simulink model "surge_tank_level_sim"  (R2021b)
settings: Solver=VariableStepAuto  StartTime=0.0  StopTime=5000  MaxStep=0.1  RelTol=1e-3  EnableMultiTasking=on
InitFcn:
  | load("mpcobj.mat")
StopFcn:
  | addpath("~/ml-plot-utils")
  | 
  | figure(1); clf
  | u_labels = ["$u(k)$" "$p(k)$"];
  | make_iorplot(y, t, [u p], r, u_labels)
  | sp1 = subplot(2,1,1);
  | ylim(sp1,axes_limits_with_margin(y, 0.1, [0 100]))
  | 
  | figure(2); clf
  | u_labels = ["$u(k)$" "$p(k)$"];
  | make_iorplot(y1, t, [u1 p], r, u_labels)
  | sp1 = subplot(2,1,1);
  | ylim(sp1,axes_limits_with_margin(y, 0.1, [0 100]))
  | 
  | figure(3); clf
  | u_labels = ["$u(k)$" "$p(k)$"];
  | make_iorplot(y2, t, [u2 p], r, u_labels)
  | sp1 = subplot(2,1,1);
  | ylim(sp1,axes_limits_with_margin(y, 0.1, [0 100]))
  | 
  | figure(4); clf
  | u_labels = ["$u(k)$" "$p(k)$"];
  | make_iorplot(y3, t, [u3 p], r, u_labels)
  | sp1 = subplot(2,1,1);
  | ylim(sp1,[0 100])
  | yline(15, '--', 'Parent', sp1)
  | yline(85, '--', 'Parent', sp1)
  | labels = sp1.Legend.String;
  | labels(3:4) = {'$y_{min}$', '$y_{max}$'};
  | set(sp1.Legend, 'String', labels)
  | 
  | figure(5); clf
  | u_labels = ["$u(k)$" "$p(k)$"];
  | make_iorplot(y4, t, [u4 p], r, u_labels)
  | sp1 = subplot(2,1,1);
  | ylim(sp1,[0 100])
  | yline(15, '--', 'Parent', sp1)
  | yline(85, '--', 'Parent', sp1)
  | labels = sp1.Legend.String;
  | labels(3:4) = {'$y_{min}$', '$y_{max}$'};
  | set(sp1.Legend, 'String', labels)
  | 
  | figure(6); clf
  | u_labels = ["$u(k)$" "$p(k)$"];
  | make_iorplot(y5, t, [u5 p], r, u_labels)
  | sp1 = subplot(2,1,1);
  | ylim(sp1,[0 100])
  | yline(15, '--', 'Parent', sp1)
  | yline(85, '--', 'Parent', sp1)
  | labels = sp1.Legend.String;
  | labels(3:4) = {'$y_{min}$', '$y_{max}$'};
  | set(sp1.Legend, 'String', labels)
  | 
  | figure(7); clf
  | u_labels = ["$u(k)$" "$p(k)$"];
  | make_iorplot(y6, t, [u6 p], r, u_labels)
  | sp1 = subplot(2,1,1);
  | ylim(sp1,[0 100])
  | yline(15,'--', 'Parent', sp1)
  | yline(85, '--', 'Parent', sp1)
  | labels = sp1.Legend.String;
  | labels(3:4) = {'$y_{min}$', '$y_{max}$'};
  | set(sp1.Legend, 'String', labels)
  | 
  | figure(7); clf
  | u_labels = ["$u(k)$" "$p(k)$"];
  | make_iorplot(y6, t, [u6 p], r, u_labels)
  | sp1 = subplot(2,1,1);
  | ylim(sp1,[0 100])
  | yline(15,'--', 'Parent', sp1)
  | yline(85, '--', 'Parent', sp1)
  | labels = sp1.Legend.String;
  | labels(3:4) = {'$y_{min}$', '$y_{max}$'};
  | set(sp1.Legend, 'String', labels)
  | 
  | figure(8); clf
  | u_labels = ["$u(k)$" "$p(k)$"];
  | make_iorplot(y7, t, [u7 p], r, u_labels)
  | sp1 = subplot(2,1,1);
  | ylim(sp1,[0 100])
  | yline(15,'--', 'Parent', sp1)
  | yline(85, '--', 'Parent', sp1)
  | labels = sp1.Legend.String;
  | labels(3:4) = {'$y_{min}$', '$y_{max}$'};
  | set(sp1.Legend, 'String', labels)
  | 
  | figure(9); clf
  | u_labels = ["$u(k)$" "$p(k)$"];
  | make_iorplot(y8, t, [u8 p], r, u_labels)
  | sp1 = subplot(2,1,1);
  | ylim(sp1,[0 100])
  | yline(15,'--', 'Parent', sp1)
  | yline(85, '--', 'Parent', sp1)
  | labels = sp1.Legend.String;
  | labels(3:4) = {'$y_{min}$', '$y_{max}$'};
  | set(sp1.Legend, 'String', labels)
undefined symbols (not defined in the file or in its folder): DiscIntNeverNeededParam
libraries: simulink x10, dspstat3 x3, mpclib x1
settings Model: PacingRate=10  Creator=Eric  LastModifiedBy=billtubbs
settings SolverCC: ZeroCrossAlgorithm=Adaptive  AlgebraicLoopSolver=TrustRegion
settings DataIOCC: LimitDataPoints=on  SaveFormat=StructureWithTime  SignalLoggingSaveFormat=ModelDataLogs  SaveTime=off  ReturnWorkspaceOutputs=off
settings OptimizationCC: ExpressionDepthLimit=2147483647  LifeSpan=inf
settings DebuggingCC: AlgebraicLoopMsg=none  UnderspecifiedInitializationDetection=Classic  MergeDetectMultiDrivingBlocksExec=none  IgnoredZcDiagnostic=none  FcnCallInpInsideContextMsg=warning  UnconnectedInputMsg=none  UnconnectedOutputMsg=none  UnconnectedLineMsg=none  StateNameClashWarn=warning  SFUnexpectedBacktrackingDiag=warning  SFNoUnconditionalDefaultTransitionDiag=warning  SFExecutionAtInitializationDiag=none  SFMachineParentedDataDiag=warning  ArithmeticOperatorsInVariantConditions=warning
settings HardwareCC: ProdBitPerPointer=32  ProdBitPerSizeT=32  ProdBitPerPtrDiffT=32  ProdLargestAtomicFloat=None  ProdIntDivRoundTo=Undefined  ProdEndianess=Unspecified  ProdWordSize=32  ProdHWDeviceType=32-bit Generic
settings ModelReferenceCC: PropagateSignalLabelsOutOfModel=off
settings SFSimCC: SimUseLocalCustomCode=off  CustomCodeUndefinedFunction=UseInterfaceOnly
settings RTWCC: RTWUseLocalCustomCode=off
settings CodeAppCC: StateflowObjectComments=on
settings GRTTargetCC: TargetLangStandard=C89/C90 (ANSI)  CombineOutputUpdateFcns=off  GRTInterface=on
settings ConfigComp: CovMetricSettings=dw  CovSaveCumulativeToWorkspaceVar=on  CovSaveSingleToWorkspaceVar=on  CovExternalEMLEnable=off  CovSFcnEnable=off

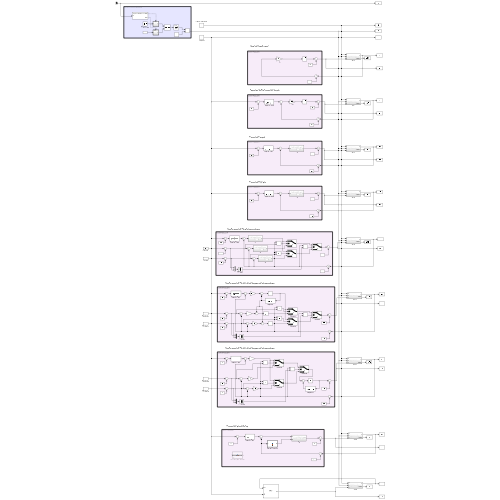
[thumbnail: Simulink's stored preview of the top-level diagram]
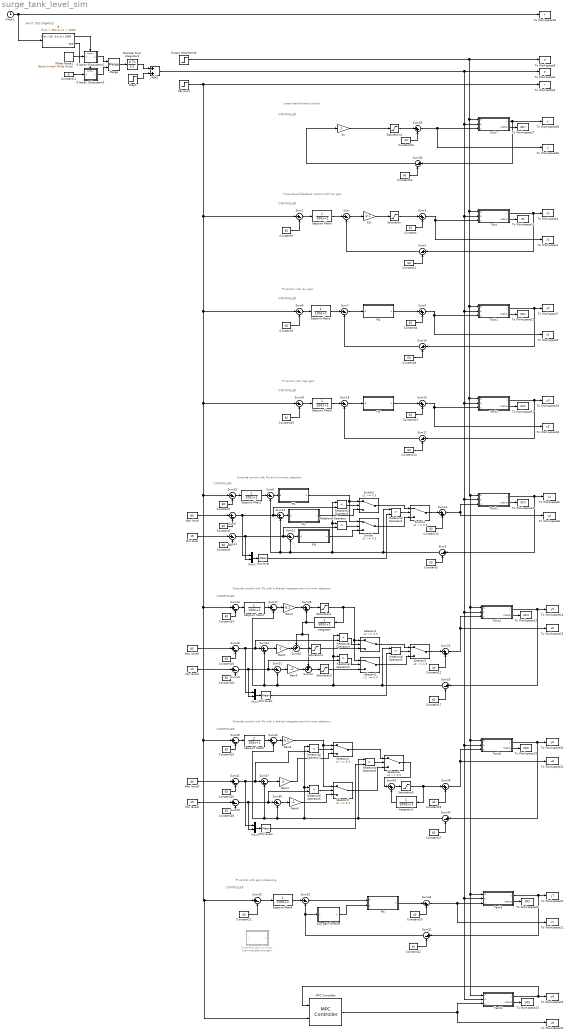
== system surge_tank_level_sim ==
  note: Proportional feedback control with low gain
  note: Override control with PIs and min-max selectors
  note: CONTROLLER
  note: CONTROLLER
  note: INPUT DISTURBANCE
  note: PI control with low gain
  note: CONTROLLER
  note: CONTROLLER
  note: PI control with high gain
  note: CONTROLLER
  note: Override control with PIs with a shared integrator and min-max selectors
  note: PI control with gain scheduling
  note: CONTROLLER
  note: CONTROLLER
  note: Linear feed-forward control
  note: CONTROLLER
  note: Override control with PIs with a shared integrator and min-max selectors
  Add1 : Sum
  Clock1 : Clock
  Constant{,4,10,12..13,20,23,25} (8 alike) : Constant  Value=40
  Constant{1..3,5..9,14..19,21..22,24,26..29} (21 alike) : Constant  Value=60
  Constant11 : Constant  Value=0
  Discrete-Time Integrator1 : DiscreteIntegrator  gainval=1  SampleTime=-1  ICPrevOutput=DiscIntNeverNeededParam  ICPrevScaledInput=DiscIntNeverNeededParam
  Exp gain function : MATLAB Function  TreatAsAtomicUnit=on
  Gain{1,3..4,6} (4 alike) : Gain  Gain=-2
  Gain2 : Gain  Gain=-0.1
  Gain5 : Gain  Gain=-0.1
  If : If  IfExpression=u1 > 500 & u1 < 1000
  If Action Subsystem2 : Subsystem  TreatAsAtomicUnit=on
  If Action Subsystem3 : Subsystem  TreatAsAtomicUnit=on
  Integrator : TransferFcn  Numerator=1  Denominator=[500 1]
  Integrator1 : TransferFcn  Numerator=1  Denominator=[1000 1]
  Kc : Gain
  Kc1 : Gain  Gain=-0.1
  MPC Controller : mpclib/MPC Controller  mpcobj=mpcobj  x0=[]  is_multiple=0  enable_value=0  return_u0=off  updateMPCinCallerWorkspace=on  md_inport=off  mv_inport=off  uref_inport=off  return_cost=off  return_mvseq=off  return_qpstatus=off  return_xseq=off  return_state=off  return_ovseq=off  state_inport=off  umin_inport=off  umax_inport=off  ymin_inport=off  ymax_inport=off  cc_inport=off  ywt_inport=off  uwt_inport=off  duwt_inport=off  rhoeps_inport=off  pm_inport=off  MaximumP=10  HorizonChoice=FixedHorizon  n_ts=5  n_p=200  n_mv=1  n_md=0  n_ud=1  n_mo=1  n_uo=0  BlockDataType=double  SampleTimeInherited=off  switch_inport=off
  Max level : Constant  Value=85
  Max level1 : Constant  Value=85
  Max level2 : Constant  Value=85
  Merge : Merge
  Mid level : dspstat3/Mean  run=off  InputProcessing=Columns as channels (frame based)  reset_popup=None  directionMode=Entire input  dimension=1  roiEnable=off  roiType=Rectangles  roiPortion=Entire ROI  roiOutput=Individual statistics for each ROI  roiFlag=off  roundingMode=Floor  overflowMode=off  outputDataTypeStr=Inherit: Same as accumulator  outputMin=[]  outputMax=[]  outputLastDataTypeStr=Inherit: Same as accumulator
  Mid level1 : dspstat3/Mean  run=off  InputProcessing=Columns as channels (frame based)  reset_popup=None  directionMode=Entire input  dimension=1  roiEnable=off  roiType=Rectangles  roiPortion=Entire ROI  roiOutput=Individual statistics for each ROI  roiFlag=off  roundingMode=Floor  overflowMode=off  outputDataTypeStr=Inherit: Same as accumulator  outputMin=[]  outputMax=[]  outputLastDataTypeStr=Inherit: Same as accumulator
  Mid level2 : dspstat3/Mean  run=off  InputProcessing=Columns as channels (frame based)  reset_popup=None  directionMode=Entire input  dimension=1  roiEnable=off  roiType=Rectangles  roiPortion=Entire ROI  roiOutput=Individual statistics for each ROI  roiFlag=off  roundingMode=Floor  overflowMode=off  outputDataTypeStr=Inherit: Same as accumulator  outputMin=[]  outputMax=[]  outputLastDataTypeStr=Inherit: Same as accumulator
  Min level : Constant  Value=15
  Min level1 : Constant  Value=15
  Min level2 : Constant  Value=15
  Mux1 : Mux  Inputs=2
  Mux2 : Mux  Inputs=2
  Mux3 : Mux  Inputs=2
  Output disturbance : Step  After=0  SampleTime=0
  PI1 : Subsystem
  PI2 : Subsystem
  PI3 : Subsystem
  PI4 : Subsystem
  PI5 : Subsystem
  PI6 : Subsystem
  Quadratic gain function : MATLAB Function  Commented=through  TreatAsAtomicUnit=on
  Relational Operator{,2..3,5..6,8} (6 alike) : RelationalOperator  Operator=>  OutDataTypeStr=boolean  RndMeth=Nearest
  Relational Operator1 : RelationalOperator  Operator=<  OutDataTypeStr=boolean  RndMeth=Nearest
  Relational Operator4 : RelationalOperator  Operator=<  OutDataTypeStr=boolean  RndMeth=Nearest
  Relational Operator7 : RelationalOperator  Operator=<  OutDataTypeStr=boolean  RndMeth=Nearest
  Saturation{,1..5} (6 alike) : Saturate  UpperLimit=60  LowerLimit=-40
  Selector{1..6} (6 alike) : Switch  Threshold=0.5
  Set point : Step  Time=100  Before=60  After=50  SampleTime=0
  Setpoint filter{0..6} (7 alike) : TransferFcn  Denominator=[100 1]
  Step1 : Step  Time=900  After=10  SampleTime=0
  Sum{,1..2,4..8,10..13,15..19,21..22,24..27,29..33,36..37,39..42} (34 alike) : Sum  Inputs=|+-
  Sum{3,9,14,20,23,28,34..35,38,43} (10 alike) : Sum  Inputs=|++
  Sum44 : Sum  Inputs=++|
  Sum45 : Sum  Inputs=++|
  Switch : Switch  Threshold=0.5
  Switch1 : Switch  Threshold=0.5
  Switch2 : Switch  Threshold=0.5
  Tank : Subsystem
  Tank1 : Subsystem
  Tank2 : Subsystem
  Tank3 : Subsystem
  Tank4 : Subsystem
  Tank5 : Subsystem
  Tank6 : Subsystem
  Tank7 : Subsystem
  Tank8 : Subsystem
  To Workspace1 : ToWorkspace  VariableName=u1  SampleTime=1
  To Workspace10 : ToWorkspace  VariableName=OF  SaveFormat=Timeseries  SampleTime=-1
  To Workspace11 : ToWorkspace  VariableName=OF1  SaveFormat=Timeseries  SampleTime=-1
  To Workspace12 : ToWorkspace  VariableName=OF3  SaveFormat=Timeseries  SampleTime=-1
  To Workspace13 : ToWorkspace  VariableName=OF4  SaveFormat=Timeseries  SampleTime=-1
  To Workspace14 : ToWorkspace  VariableName=y5  SampleTime=1
  To Workspace15 : ToWorkspace  VariableName=u5  SampleTime=1
  To Workspace16 : ToWorkspace  VariableName=t  SampleTime=1
  To Workspace17 : ToWorkspace  VariableName=OF2  SaveFormat=Timeseries  SampleTime=-1
  To Workspace18 : ToWorkspace  VariableName=u3  SampleTime=1
  To Workspace19 : ToWorkspace  VariableName=y3  SampleTime=1
  To Workspace2 : ToWorkspace  VariableName=y1  SampleTime=1
  To Workspace20 : ToWorkspace  VariableName=OF5  SaveFormat=Timeseries  SampleTime=-1
  To Workspace21 : ToWorkspace  VariableName=u7  SampleTime=1
  To Workspace22 : ToWorkspace  VariableName=y7  SampleTime=1
  To Workspace23 : ToWorkspace  VariableName=OF6  SaveFormat=Timeseries  SampleTime=-1
  To Workspace24 : ToWorkspace  VariableName=u8  SampleTime=1
  To Workspace25 : ToWorkspace  VariableName=y8  SampleTime=1
  To Workspace26 : ToWorkspace  VariableName=u  SampleTime=1
  To Workspace27 : ToWorkspace  VariableName=OF7  SaveFormat=Timeseries  SampleTime=-1
  To Workspace28 : ToWorkspace  VariableName=y  SampleTime=1
  To Workspace29 : ToWorkspace  VariableName=OF8  SaveFormat=Timeseries  SampleTime=-1
  To Workspace3 : ToWorkspace  VariableName=r  SampleTime=1
  To Workspace30 : ToWorkspace  VariableName=y6  SampleTime=1
  To Workspace31 : ToWorkspace  VariableName=u6  SampleTime=1
  To Workspace4 : ToWorkspace  VariableName=p  SampleTime=1
  To Workspace5 : ToWorkspace  VariableName=u2  SampleTime=1
  To Workspace6 : ToWorkspace  VariableName=y4  SampleTime=1
  To Workspace7 : ToWorkspace  VariableName=y2  SampleTime=1
  To Workspace8 : ToWorkspace  VariableName=u4  SampleTime=1
  To Workspace9 : ToWorkspace  VariableName=d  SampleTime=1
  White Noise1 : simulink/Sources/Band-Limited White Noise  Cov=0.1  Ts=1  seed=[10000]
  wires:
  Setpoint filter2/1 -> Sum6/1
  Sum2/1 -> Relational Operator1/1, Relational Operator/1, Sum12/2, Sum13/2, Sum6/2, Relational Operator2/1
  Sum6/1 -> PI1/1(e)
  PI1/1(u) -> Switch/1, Switch1/1
  Sum5/1 -> Relational Operator1/2, Sum13/1, Mux1/1
  Relational Operator1/1 -> Switch1/2
  Sum13/1 -> PI2/1(e)
  Sum12/1 -> PI3/1(e)
  Sum11/1 -> Relational Operator/2, Sum12/1, Mux1/2
  Relational Operator/1 -> Switch/2
  PI2/1(u) -> Switch1/3
  PI3/1(u) -> Switch/3
  Switch1/1 -> Switch2/1
  Switch/1 -> Switch2/3
  Relational Operator2/1 -> Switch2/2
  Mid level/1 -> Relational Operator2/2
  Constant2/1 -> Sum5/2
  Max level/1 -> Sum5/1
  Constant5/1 -> Sum11/2
  Min level/1 -> Sum11/1
  Sum15/1 -> Setpoint filter2/1
  Constant7/1 -> Sum15/2
  Mux1/1 -> Mid level/1
  Sum4/1 -> Sum/2
  Constant6/1 -> Sum1/2
  Sum3/1 -> To Workspace1/1, Tank/3(u)
  Tank/1(y) -> Sum4/1, To Workspace2/1
  Tank/2(status) -> To Workspace10/1
  Constant1/1 -> Sum4/2
  Constant/1 -> Sum3/2
  Sum/1 -> Kc1/1
  Saturation/1 -> Sum3/1
  Constant3/1 -> Sum2/2
  Sum14/1 -> Tank2/3(u), To Workspace8/1
  Tank2/2(status) -> To Workspace12/1
  Tank2/1(y) -> Sum2/1, To Workspace6/1
  Kc1/1 -> Saturation/1
  Sum8/1 -> Setpoint filter1/1
  Tank1/1(y) -> Sum10/1, To Workspace7/1
  Sum7/1 -> PI4/1(e)
  PI4/1(u) -> Sum9/1
  Constant8/1 -> Sum10/2
  Setpoint filter1/1 -> Sum7/1
  Tank1/2(status) -> To Workspace11/1
  Sum9/1 -> Tank1/3(u), To Workspace5/1
  Constant4/1 -> Sum9/2
  Constant9/1 -> Sum8/2
  If/1 -> If Action Subsystem2/Action
  If/2 -> If Action Subsystem3/Action
  Clock1/1 -> If/1, To Workspace16/1
  If Action Subsystem2/1(Out1) -> Merge/1
  If Action Subsystem3/1(Out1) -> Merge/2
  White Noise1/1 -> If Action Subsystem2/1(In1)
  Constant11/1 -> If Action Subsystem3/1(In1)
  Discrete-Time Integrator1/1 -> Add1/1
  Step1/1 -> Add1/2
  Merge/1 -> Discrete-Time Integrator1/1
  Constant10/1 -> Sum14/2
  Switch2/1 -> Sum14/1
  Sum1/1 -> Setpoint filter0/1
  Setpoint filter0/1 -> Sum/1
  Sum10/1 -> Sum7/2
  Tank3/1(y) -> Sum17/1, To Workspace19/1
  Add1/1 -> Tank3/2(p), Tank4/2(p), Tank8/2(p), Tank5/2(p), Tank6/2(p), Tank2/2(p), Tank1/2(p), Tank/2(p), Tank7/2(p), To Workspace4/1
  PI5/1(u) -> Sum20/1
  Constant14/1 -> Sum17/2
  Constant15/1 -> Sum19/2
  Sum18/1 -> PI5/1(e)
  Sum20/1 -> Tank3/3(u), To Workspace18/1
  Constant13/1 -> Sum20/2
  Output disturbance/1 -> Tank/1(d), Tank3/1(d), Tank4/1(d), Tank8/1(d), Tank5/1(d), Tank6/1(d), Tank2/1(d), Tank1/1(d), Tank7/1(d), To Workspace9/1
  Sum17/1 -> Sum18/2
  Tank3/2(status) -> To Workspace17/1
  Sum19/1 -> Setpoint filter5/1
  Sum23/1 -> To Workspace15/1, Tank4/3(u)
  Mux2/1 -> Mid level1/1
  Constant16/1 -> Sum26/2
  Tank4/2(status) -> To Workspace13/1
  Selector1/1 -> Selector3/1
  Selector2/1 -> Selector3/3
  Saturation2/1 -> Selector1/3
  Sum26/1 -> Relational Operator4/2, Sum22/1, Mux2/1
  Constant18/1 -> Sum16/2
  Saturation3/1 -> Selector2/3
  Constant12/1 -> Sum23/2
  Constant17/1 -> Sum25/2
  Sum25/1 -> Sum27/2, Sum22/2, Sum21/2, Relational Operator3/1, Relational Operator4/1, Relational Operator5/1
  Relational Operator3/1 -> Selector2/2
  Setpoint filter3/1 -> Sum27/1
  Max level1/1 -> Sum26/1
  Constant19/1 -> Sum24/2
  Min level1/1 -> Sum16/1
  Mid level1/1 -> Relational Operator5/2
  Relational Operator5/1 -> Selector3/2
  Gain2/1 -> Sum28/1
  Tank4/1(y) -> Sum25/1, To Workspace14/1
  Sum24/1 -> Setpoint filter3/1
  Relational Operator4/1 -> Selector1/2
  Sum16/1 -> Sum21/1, Relational Operator3/2, Mux2/2
  Sum27/1 -> Gain2/1
  Gain1/1 -> Sum45/2
  Gain3/1 -> Sum44/2
  Sum22/1 -> Gain1/1
  Constant20/1 -> Sum34/2
  PI6/1(u) -> Sum34/1
  Tank5/2(status) -> To Workspace20/1
  Tank5/1(y) -> Sum31/1, To Workspace22/1
  Sum34/1 -> To Workspace21/1, Tank5/3(u)
  Sum33/1 -> Setpoint filter4/1
  Sum31/1 -> Sum32/2, Exp gain function/1(y)
  Constant21/1 -> Sum33/2
  Constant22/1 -> Sum31/2
  Sum32/1 -> PI6/1(e)
  Setpoint filter4/1 -> Sum32/1
  Exp gain function/1(K) -> PI6/2(K)
  Tank6/2(status) -> To Workspace23/1
  Tank6/1(y) -> MPC Controller/1, To Workspace25/1
  MPC Controller/1 -> To Workspace24/1, Tank6/3(u)
  Tank7/2(status) -> To Workspace27/1
  Kc/1 -> Saturation4/1
  Sum35/1 -> To Workspace26/1, Tank7/3(u)
  Tank7/1(y) -> Sum36/1, To Workspace28/1
  Constant24/1 -> Sum36/2
  Constant23/1 -> Sum35/2
  Saturation4/1 -> Sum35/1
  Sum36/1 -> Kc/1
  Setpoint filter5/1 -> Sum18/1
  Sum28/1 -> Saturation1/1
  Saturation1/1 -> Integrator/1, Selector1/1, Selector2/1
  Integrator/1 -> Sum44/1, Sum45/1, Sum28/2
  Sum21/1 -> Gain3/1
  Tank8/2(status) -> To Workspace29/1
  Sum37/1 -> Gain4/1
  Set point/1 -> Sum1/1, Sum19/1, Sum15/1, Sum24/1, Sum39/1, MPC Controller/2, Sum33/1, Sum8/1, To Workspace3/1
  Sum40/1 -> Sum42/2, Sum37/2, Sum30/2, Relational Operator7/1, Relational Operator6/1, Relational Operator8/1
  Selector5/1 -> Selector6/3
  Sum41/1 -> Relational Operator7/2, Sum37/1, Mux3/1
  Relational Operator7/1 -> Selector4/2
  Gain4/1 -> Selector4/3
  Sum42/1 -> Gain5/1
  Gain6/1 -> Selector5/3
  Constant28/1 -> Sum29/2
  Constant27/1 -> Sum40/2
  Constant29/1 -> Sum39/2
  Mid level2/1 -> Relational Operator8/2
  Max level2/1 -> Sum41/1
  Gain5/1 -> Selector5/1, Selector4/1
  Constant25/1 -> Sum38/2
  Setpoint filter6/1 -> Sum42/1
  Sum29/1 -> Sum30/1, Relational Operator6/2, Mux3/2
  Min level2/1 -> Sum29/1
  Sum38/1 -> To Workspace31/1, Tank8/3(u)
  Tank8/1(y) -> Sum40/1, To Workspace30/1
  Mux3/1 -> Mid level2/1
  Sum39/1 -> Setpoint filter6/1
  Relational Operator6/1 -> Selector5/2
  Selector6/1 -> Sum43/1
  Selector4/1 -> Selector6/1
  Sum43/1 -> Saturation5/1
  Saturation5/1 -> Sum38/1, Integrator1/1
  Relational Operator8/1 -> Selector6/2
  Integrator1/1 -> Sum43/2
  Constant26/1 -> Sum41/2
  Sum30/1 -> Gain6/1
  Selector3/1 -> Sum23/1
  Sum45/1 -> Saturation2/1
  Sum44/1 -> Saturation3/1

== system surge_tank_level_sim/If Action Subsystem2 ==
  In1 : Inport
  Action Port : ActionPort  ActionPortLabel=if(u1 > 500 & u1 < 1000)
  Out1 : Outport
  wires:
  In1/1 -> Out1/1

== system surge_tank_level_sim/If Action Subsystem3 ==
  In1 : Inport
  Action Port : ActionPort  ActionPortLabel=else
  Out1 : Outport
  wires:
  In1/1 -> Out1/1

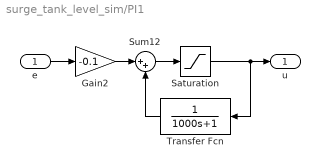
== system surge_tank_level_sim/PI1 ==
  e : Inport
  Gain2 : Gain  Gain=-0.1
  Saturation : Saturate  UpperLimit=60  LowerLimit=-40
  Sum12 : Sum  Inputs=|++
  Transfer Fcn : TransferFcn  Numerator=1  Denominator=[1000 1]
  u : Outport
  wires:
  e/1 -> Gain2/1
  Transfer Fcn/1 -> Sum12/2
  Gain2/1 -> Sum12/1
  Sum12/1 -> Saturation/1
  Saturation/1 -> Transfer Fcn/1, u/1

== system surge_tank_level_sim/PI2 ==
  e : Inport
  Gain2 : Gain  Gain=-2
  Saturation : Saturate  UpperLimit=60  LowerLimit=-40
  Sum12 : Sum  Inputs=|++
  Transfer Fcn : TransferFcn  Numerator=1  Denominator=[40 1]
  u : Outport
  wires:
  e/1 -> Gain2/1
  Transfer Fcn/1 -> Sum12/2
  Gain2/1 -> Sum12/1
  Sum12/1 -> Saturation/1
  Saturation/1 -> Transfer Fcn/1, u/1

== system surge_tank_level_sim/PI3 ==
  e : Inport
  Gain2 : Gain  Gain=-2
  Saturation : Saturate  UpperLimit=60  LowerLimit=-40
  Sum12 : Sum  Inputs=|++
  Transfer Fcn : TransferFcn  Numerator=1  Denominator=[40 1]
  u : Outport
  wires:
  e/1 -> Gain2/1
  Transfer Fcn/1 -> Sum12/2
  Gain2/1 -> Sum12/1
  Sum12/1 -> Saturation/1
  Saturation/1 -> Transfer Fcn/1, u/1

== system surge_tank_level_sim/PI4 ==
  e : Inport
  Gain2 : Gain  Gain=-0.1
  Saturation : Saturate  UpperLimit=60  LowerLimit=-40
  Sum12 : Sum  Inputs=|++
  Transfer Fcn : TransferFcn  Numerator=1  Denominator=[1000 1]
  u : Outport
  wires:
  e/1 -> Gain2/1
  Transfer Fcn/1 -> Sum12/2
  Gain2/1 -> Sum12/1
  Sum12/1 -> Saturation/1
  Saturation/1 -> Transfer Fcn/1, u/1

== system surge_tank_level_sim/PI5 ==
  e : Inport
  Gain2 : Gain  Gain=-2
  Saturation : Saturate  UpperLimit=60  LowerLimit=-40
  Sum12 : Sum  Inputs=|++
  Transfer Fcn : TransferFcn  Numerator=1  Denominator=[40 1]
  u : Outport
  wires:
  e/1 -> Gain2/1
  Transfer Fcn/1 -> Sum12/2
  Gain2/1 -> Sum12/1
  Sum12/1 -> Saturation/1
  Saturation/1 -> Transfer Fcn/1, u/1

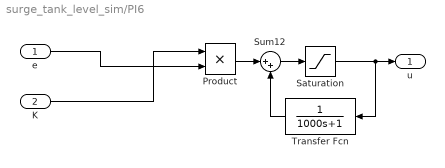
== system surge_tank_level_sim/PI6 ==
  e : Inport
  K : Inport  Port=2
  Product : Product
  Saturation : Saturate  UpperLimit=60  LowerLimit=-40
  Sum12 : Sum  Inputs=|++
  Transfer Fcn : TransferFcn  Numerator=1  Denominator=[1000 1]
  u : Outport
  wires:
  e/1 -> Product/2
  Transfer Fcn/1 -> Sum12/2
  Product/1 -> Sum12/1
  Sum12/1 -> Saturation/1
  Saturation/1 -> Transfer Fcn/1, u/1
  K/1 -> Product/1

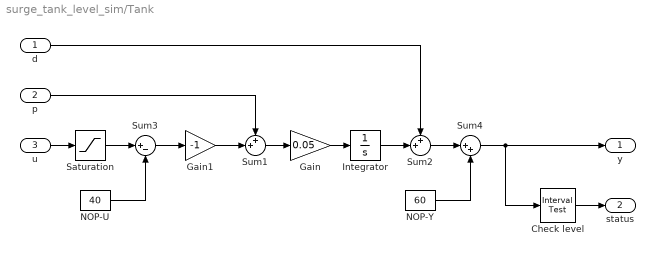
== system surge_tank_level_sim/Tank ==
  d : Inport
  p : Inport  Port=2
  u : Inport  Port=3
  Check level : simulink/Logic and Bit Operations/Interval Test  IntervalClosedRight=on  uplimit=100  IntervalClosedLeft=on  lowlimit=0  OutDataTypeStr=boolean
  Gain : Gain  Gain=0.05
  Gain1 : Gain  Gain=-1
  Integrator : Integrator
  NOP-U : Constant  Value=40
  NOP-Y : Constant  Value=60
  Saturation : Saturate  UpperLimit=100  LowerLimit=0
  Sum1 : Sum  Inputs=++|
  Sum2 : Sum  Inputs=++|
  Sum3 : Sum  Inputs=|+-
  Sum4 : Sum  Inputs=|++
  y : Outport
  status : Outport  Port=2
  wires:
  d/1 -> Sum2/1
  Gain/1 -> Integrator/1
  p/1 -> Sum1/1
  Integrator/1 -> Sum2/2
  Sum2/1 -> Sum4/1
  u/1 -> Saturation/1
  Sum1/1 -> Gain/1
  NOP-U/1 -> Sum3/2
  NOP-Y/1 -> Sum4/2
  Sum4/1 -> y/1, Check level/1
  Check level/1 -> status/1
  Saturation/1 -> Sum3/1
  Gain1/1 -> Sum1/2
  Sum3/1 -> Gain1/1

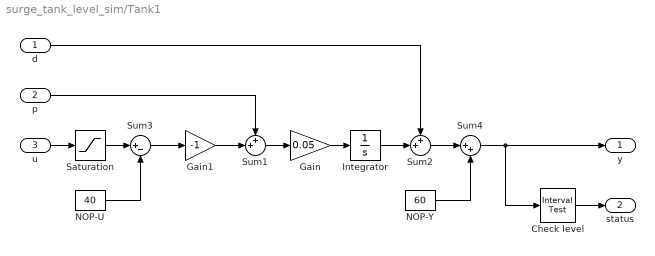
== system surge_tank_level_sim/Tank1 ==
  d : Inport
  p : Inport  Port=2
  u : Inport  Port=3
  Check level : simulink/Logic and Bit Operations/Interval Test  IntervalClosedRight=on  uplimit=100  IntervalClosedLeft=on  lowlimit=0  OutDataTypeStr=boolean
  Gain : Gain  Gain=0.05
  Gain1 : Gain  Gain=-1
  Integrator : Integrator
  NOP-U : Constant  Value=40
  NOP-Y : Constant  Value=60
  Saturation : Saturate  UpperLimit=100  LowerLimit=0
  Sum1 : Sum  Inputs=++|
  Sum2 : Sum  Inputs=++|
  Sum3 : Sum  Inputs=|+-
  Sum4 : Sum  Inputs=|++
  y : Outport
  status : Outport  Port=2
  wires:
  d/1 -> Sum2/1
  Gain/1 -> Integrator/1
  p/1 -> Sum1/1
  Integrator/1 -> Sum2/2
  Sum2/1 -> Sum4/1
  u/1 -> Saturation/1
  Sum1/1 -> Gain/1
  NOP-U/1 -> Sum3/2
  NOP-Y/1 -> Sum4/2
  Sum4/1 -> y/1, Check level/1
  Check level/1 -> status/1
  Saturation/1 -> Sum3/1
  Gain1/1 -> Sum1/2
  Sum3/1 -> Gain1/1

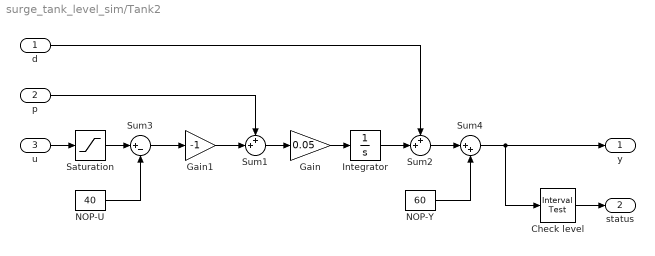
== system surge_tank_level_sim/Tank2 ==
  d : Inport
  p : Inport  Port=2
  u : Inport  Port=3
  Check level : simulink/Logic and Bit Operations/Interval Test  IntervalClosedRight=on  uplimit=100  IntervalClosedLeft=on  lowlimit=0  OutDataTypeStr=boolean
  Gain : Gain  Gain=0.05
  Gain1 : Gain  Gain=-1
  Integrator : Integrator
  NOP-U : Constant  Value=40
  NOP-Y : Constant  Value=60
  Saturation : Saturate  UpperLimit=100  LowerLimit=0
  Sum1 : Sum  Inputs=++|
  Sum2 : Sum  Inputs=++|
  Sum3 : Sum  Inputs=|+-
  Sum4 : Sum  Inputs=|++
  y : Outport
  status : Outport  Port=2
  wires:
  d/1 -> Sum2/1
  Gain/1 -> Integrator/1
  p/1 -> Sum1/1
  Integrator/1 -> Sum2/2
  Sum2/1 -> Sum4/1
  u/1 -> Saturation/1
  Sum1/1 -> Gain/1
  NOP-U/1 -> Sum3/2
  NOP-Y/1 -> Sum4/2
  Sum4/1 -> y/1, Check level/1
  Check level/1 -> status/1
  Saturation/1 -> Sum3/1
  Gain1/1 -> Sum1/2
  Sum3/1 -> Gain1/1

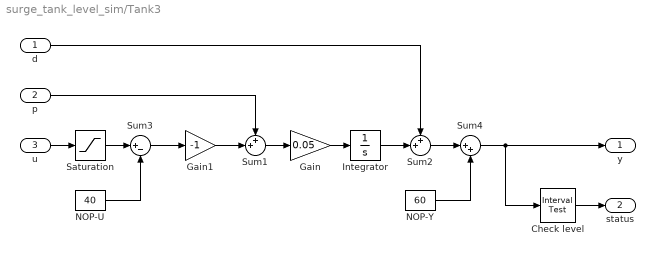
== system surge_tank_level_sim/Tank3 ==
  d : Inport
  p : Inport  Port=2
  u : Inport  Port=3
  Check level : simulink/Logic and Bit Operations/Interval Test  IntervalClosedRight=on  uplimit=100  IntervalClosedLeft=on  lowlimit=0  OutDataTypeStr=boolean
  Gain : Gain  Gain=0.05
  Gain1 : Gain  Gain=-1
  Integrator : Integrator
  NOP-U : Constant  Value=40
  NOP-Y : Constant  Value=60
  Saturation : Saturate  UpperLimit=100  LowerLimit=0
  Sum1 : Sum  Inputs=++|
  Sum2 : Sum  Inputs=++|
  Sum3 : Sum  Inputs=|+-
  Sum4 : Sum  Inputs=|++
  y : Outport
  status : Outport  Port=2
  wires:
  d/1 -> Sum2/1
  Gain/1 -> Integrator/1
  p/1 -> Sum1/1
  Integrator/1 -> Sum2/2
  Sum2/1 -> Sum4/1
  u/1 -> Saturation/1
  Sum1/1 -> Gain/1
  NOP-U/1 -> Sum3/2
  NOP-Y/1 -> Sum4/2
  Sum4/1 -> y/1, Check level/1
  Check level/1 -> status/1
  Saturation/1 -> Sum3/1
  Gain1/1 -> Sum1/2
  Sum3/1 -> Gain1/1

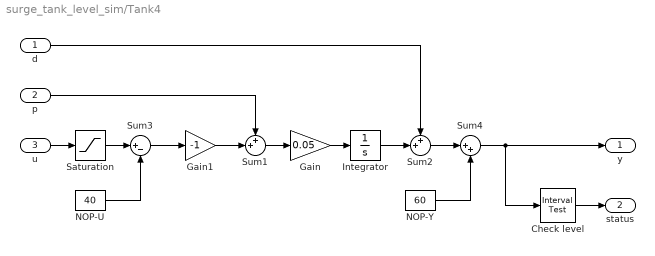
== system surge_tank_level_sim/Tank4 ==
  d : Inport
  p : Inport  Port=2
  u : Inport  Port=3
  Check level : simulink/Logic and Bit Operations/Interval Test  IntervalClosedRight=on  uplimit=100  IntervalClosedLeft=on  lowlimit=0  OutDataTypeStr=boolean
  Gain : Gain  Gain=0.05
  Gain1 : Gain  Gain=-1
  Integrator : Integrator
  NOP-U : Constant  Value=40
  NOP-Y : Constant  Value=60
  Saturation : Saturate  UpperLimit=100  LowerLimit=0
  Sum1 : Sum  Inputs=++|
  Sum2 : Sum  Inputs=++|
  Sum3 : Sum  Inputs=|+-
  Sum4 : Sum  Inputs=|++
  y : Outport
  status : Outport  Port=2
  wires:
  d/1 -> Sum2/1
  Gain/1 -> Integrator/1
  p/1 -> Sum1/1
  Integrator/1 -> Sum2/2
  Sum2/1 -> Sum4/1
  u/1 -> Saturation/1
  Sum1/1 -> Gain/1
  NOP-U/1 -> Sum3/2
  NOP-Y/1 -> Sum4/2
  Sum4/1 -> y/1, Check level/1
  Check level/1 -> status/1
  Saturation/1 -> Sum3/1
  Gain1/1 -> Sum1/2
  Sum3/1 -> Gain1/1

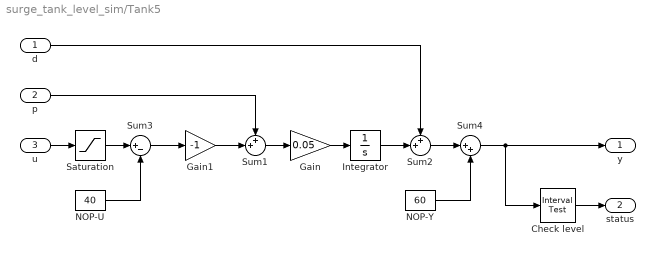
== system surge_tank_level_sim/Tank5 ==
  d : Inport
  p : Inport  Port=2
  u : Inport  Port=3
  Check level : simulink/Logic and Bit Operations/Interval Test  IntervalClosedRight=on  uplimit=100  IntervalClosedLeft=on  lowlimit=0  OutDataTypeStr=boolean
  Gain : Gain  Gain=0.05
  Gain1 : Gain  Gain=-1
  Integrator : Integrator
  NOP-U : Constant  Value=40
  NOP-Y : Constant  Value=60
  Saturation : Saturate  UpperLimit=100  LowerLimit=0
  Sum1 : Sum  Inputs=++|
  Sum2 : Sum  Inputs=++|
  Sum3 : Sum  Inputs=|+-
  Sum4 : Sum  Inputs=|++
  y : Outport
  status : Outport  Port=2
  wires:
  d/1 -> Sum2/1
  Gain/1 -> Integrator/1
  p/1 -> Sum1/1
  Integrator/1 -> Sum2/2
  Sum2/1 -> Sum4/1
  u/1 -> Saturation/1
  Sum1/1 -> Gain/1
  NOP-U/1 -> Sum3/2
  NOP-Y/1 -> Sum4/2
  Sum4/1 -> y/1, Check level/1
  Check level/1 -> status/1
  Saturation/1 -> Sum3/1
  Gain1/1 -> Sum1/2
  Sum3/1 -> Gain1/1

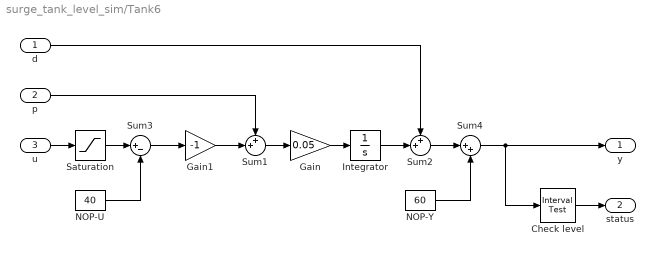
== system surge_tank_level_sim/Tank6 ==
  d : Inport
  p : Inport  Port=2
  u : Inport  Port=3
  Check level : simulink/Logic and Bit Operations/Interval Test  IntervalClosedRight=on  uplimit=100  IntervalClosedLeft=on  lowlimit=0  OutDataTypeStr=boolean
  Gain : Gain  Gain=0.05
  Gain1 : Gain  Gain=-1
  Integrator : Integrator
  NOP-U : Constant  Value=40
  NOP-Y : Constant  Value=60
  Saturation : Saturate  UpperLimit=100  LowerLimit=0
  Sum1 : Sum  Inputs=++|
  Sum2 : Sum  Inputs=++|
  Sum3 : Sum  Inputs=|+-
  Sum4 : Sum  Inputs=|++
  y : Outport
  status : Outport  Port=2
  wires:
  d/1 -> Sum2/1
  Gain/1 -> Integrator/1
  p/1 -> Sum1/1
  Integrator/1 -> Sum2/2
  Sum2/1 -> Sum4/1
  u/1 -> Saturation/1
  Sum1/1 -> Gain/1
  NOP-U/1 -> Sum3/2
  NOP-Y/1 -> Sum4/2
  Sum4/1 -> y/1, Check level/1
  Check level/1 -> status/1
  Saturation/1 -> Sum3/1
  Gain1/1 -> Sum1/2
  Sum3/1 -> Gain1/1

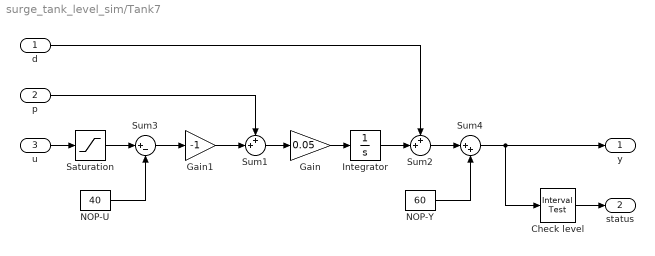
== system surge_tank_level_sim/Tank7 ==
  d : Inport
  p : Inport  Port=2
  u : Inport  Port=3
  Check level : simulink/Logic and Bit Operations/Interval Test  IntervalClosedRight=on  uplimit=100  IntervalClosedLeft=on  lowlimit=0  OutDataTypeStr=boolean
  Gain : Gain  Gain=0.05
  Gain1 : Gain  Gain=-1
  Integrator : Integrator
  NOP-U : Constant  Value=40
  NOP-Y : Constant  Value=60
  Saturation : Saturate  UpperLimit=100  LowerLimit=0
  Sum1 : Sum  Inputs=++|
  Sum2 : Sum  Inputs=++|
  Sum3 : Sum  Inputs=|+-
  Sum4 : Sum  Inputs=|++
  y : Outport
  status : Outport  Port=2
  wires:
  d/1 -> Sum2/1
  Gain/1 -> Integrator/1
  p/1 -> Sum1/1
  Integrator/1 -> Sum2/2
  Sum2/1 -> Sum4/1
  u/1 -> Saturation/1
  Sum1/1 -> Gain/1
  NOP-U/1 -> Sum3/2
  NOP-Y/1 -> Sum4/2
  Sum4/1 -> y/1, Check level/1
  Check level/1 -> status/1
  Saturation/1 -> Sum3/1
  Gain1/1 -> Sum1/2
  Sum3/1 -> Gain1/1

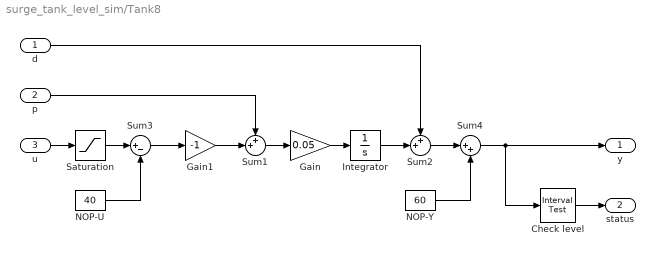
== system surge_tank_level_sim/Tank8 ==
  d : Inport
  p : Inport  Port=2
  u : Inport  Port=3
  Check level : simulink/Logic and Bit Operations/Interval Test  IntervalClosedRight=on  uplimit=100  IntervalClosedLeft=on  lowlimit=0  OutDataTypeStr=boolean
  Gain : Gain  Gain=0.05
  Gain1 : Gain  Gain=-1
  Integrator : Integrator
  NOP-U : Constant  Value=40
  NOP-Y : Constant  Value=60
  Saturation : Saturate  UpperLimit=100  LowerLimit=0
  Sum1 : Sum  Inputs=++|
  Sum2 : Sum  Inputs=++|
  Sum3 : Sum  Inputs=|+-
  Sum4 : Sum  Inputs=|++
  y : Outport
  status : Outport  Port=2
  wires:
  d/1 -> Sum2/1
  Gain/1 -> Integrator/1
  p/1 -> Sum1/1
  Integrator/1 -> Sum2/2
  Sum2/1 -> Sum4/1
  u/1 -> Saturation/1
  Sum1/1 -> Gain/1
  NOP-U/1 -> Sum3/2
  NOP-Y/1 -> Sum4/2
  Sum4/1 -> y/1, Check level/1
  Check level/1 -> status/1
  Saturation/1 -> Sum3/1
  Gain1/1 -> Sum1/2
  Sum3/1 -> Gain1/1

== matlab function surge_tank_level_sim/Exp gain function ==
  data: y input; K output
function K = fcn(y)
% Exponential function for gain scheduling of the form
%
%   gain = a + b .* (exp(-y ./ c) + exp((y - y_max) ./ c));
%
% Where a, b, and c are constants.
%
% Requirements:
% At y = 0, gain = -5
% At y = 50, gain = -0.1
% At y = 100, gain = -5
%
% Therefore:
%  a = -0.1;
%  b = -4.9;
%  c = 5;
%
% Note: normal operating point, which is 60, must
%   be added to y in this formula.
%

    K = -0.1 - 4.9 .* (exp(-(y + 60) ./ 5) + exp((y - 40) ./ 5));

end

== matlab function surge_tank_level_sim/Quadratic gain function ==
  data: y input; K output
function K = fcn(y)
% Quadratic function for gain scheduling of the form
%
%   gain = a + b * (y - 50) ^ 2
%
% Where a and b are constants.
%
% Requirements:
% At y = 0, gain = -2
% At y = 50, gain = -0.1
% At y = 100, gain = -2
%
% Therefore, a = -0.1, b = -0.00076.
%
% Solution:
% >> syms x b
% >> solve(subs(-0.1 + b * (x - 50).^2, x, 0) == -2, b)
%
% Note: normal operating point, which is 60, must
%   be added to y in this formula.
%

    K = -0.1 - 0.00076.*(y + 10).^2;

end
